simulink model "dabGAM"  (R2024b)
settings: Solver=ode23t  StartTime=0.0  StopTime=Tsim  MaxStep=dtMax  RelTol=1e-4
model workspace (MAT data in the model file):
  Cin_2 = 1e-05
  Cout_2 = 0.005
  Goff_2 = 1e-08
  L_3 = 0.001
  Lt_2 = 1e-05
  N_2 = 11
  R_1 = 0.001
  R_3 = 10
  Rds_2 = 1e-06
  Rt_2 = 0.1
  Tsim = 0.07
  Tstep = 0.035
  Vf_2 = 1e-05
  dtMax = 1e-07
  fs_2 = 50000
  order_2 = 5
libraries: nesl_utility x6, fl_lib x3, ODEsim x3
settings Model: SimulationMode=accelerator  Creator=cao2851  LastModifiedBy=cao2851
settings DataIOCC: ExternalInput=ds{1}  LoadExternalInput=on

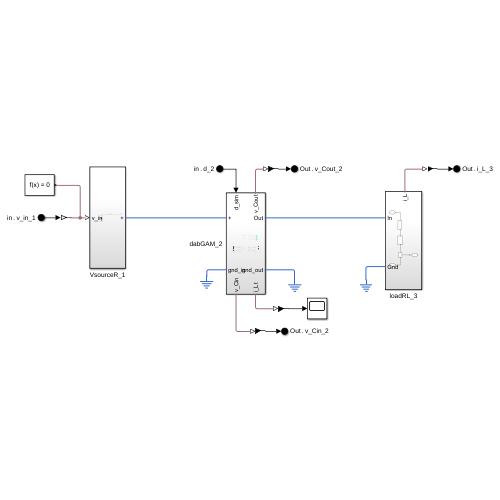
[thumbnail: Simulink's stored preview of the top-level diagram]
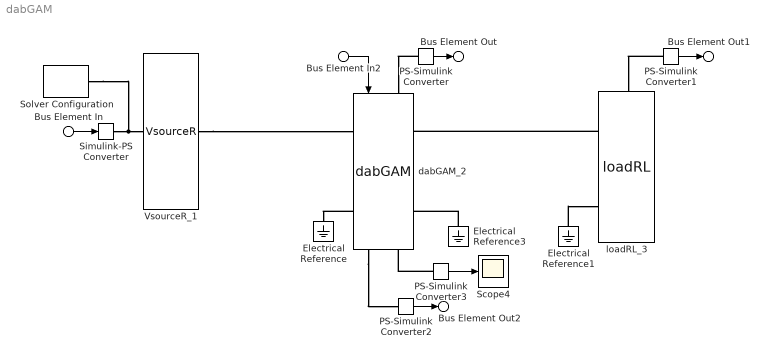
== system dabGAM ==
  Bus Element In : Inport  PortName=in  Element=v_in_1
  Bus Element In2 : Inport  PortName=in  Element=d_2
  Electrical Reference : fl_lib/Electrical/Electrical Elements/Electrical Reference
  Electrical Reference1 : fl_lib/Electrical/Electrical Elements/Electrical Reference
  Electrical Reference3 : fl_lib/Electrical/Electrical Elements/Electrical Reference
  PS-Simulink Converter{,1..3} (4 alike) : nesl_utility/PS-Simulink Converter  PhysicalDomain=network_engine_domain  SubClassName=ps_output  LeftPortType=input  RightPortType=output  PseudoPeriodic=off  Frequencies=[]  VectorFormat=inherit  Unit=inherit  AffineConversion=off
  Scope4 : Scope
  Simulink-PS Converter : nesl_utility/Simulink-PS Converter  PhysicalDomain=network_engine_domain  SubClassName=ps_input  LeftPortType=input  RightPortType=output  PseudoPeriodic=off  Frequencies=[]  NoiseDistribution=none  NoiseParameters=[]  Unit=1  AffineConversion=off  FilteringAndDerivatives=zero  SimscapeFilterOrder=1  InputFilterTimeConstant=0.001  UdotUserProvided=0
  Solver Configuration : nesl_utility/Solver Configuration  PhysicalDomain=network_engine_domain  SubClassName=solver  LeftPortType=input  RightPortType=generic  Tones=[]  Harmonics=[]  SimulateNoise=off  Profile=off  UseLocalSampling=off  EnableSwitchedLinearOptims=on  FrequencyDomain=off  UseCCode=off  RelTol=0.001  AbsTol=0.001  MinStep=1e-09  ToWorkspace=off  RevertToSquareIcSolve=off  NumHomotopyIterations=100  PhasorMode=off  PhasorModeNumHarmonics=1  ConsistencySolver=NEWTON_XTOL_AFTER_FTOL  IndexReductionMethod=DerivativeReplacement  DoDC=off  ResidualTolerance=1e-09  ConsistencyTolSource=GLOBAL  ConsistencyAbsTol=0.001  ConsistencyRelTol=0.001  ConsistencyTolFactor=1e-9  UseLocalSolver=off  LocalSolverChoice=NE_BACKWARD_EULER_ADVANCER  ResolveIndetEquations=on  FunctionEvalNumThread=1  LocalSolverSampleTime=dtMax  DoFixedCost=off  MaxNonlinIter=3  MaxModeIter=2  ComputeImpulses=off  ImpulseIterations=2  LinearAlgebra=auto  LinearAlgebraNumThread=0  EquationFormulation=NE_TIME_EF  DelaysMemoryBudget=1024  AutomaticFiltering=on  FilteringTimeConstant=0.001  PartitionStorageMethod=AS_NEEDED  PartitionMemoryBudget=1024  PartitionMethod=ROBUST  MultibodyUseLocalSolver=off  MultibodyLocalSolverChoice=ODE1  MultibodyLocalSolverSampleTime=0.001
  VsourceR_1 : ODEsim/VsourceR  SystemSampleTime=-1  VariantActivationTime=update diagram  AllowFlexibleInterface=on  Latency=0  AutoFrameSizeCalculation=off
      link override esr: R=R_1
  dabGAM_2 : ODEsim/dabGAM  SystemSampleTime=-1  VariantActivationTime=update diagram  AllowFlexibleInterface=on  Latency=0  AutoFrameSizeCalculation=off
      link override Cin: c=Cin_2
      link override Cout: C=Cout_2*10
      link override Lt: l=Lt_2  r=Rt_2
      link override S1: Rds=Rds_2  Goff=Goff_2  diode_Goff=Goff_2  diode_Ron=Rds_2  diode_Vf=Vf_2
      link override S2: Rds=Rds_2  Goff=Goff_2  diode_Goff=Goff_2  diode_Ron=Rds_2  diode_Vf=Vf_2
      link override S3: Rds=Rds_2  Goff=Goff_2  diode_Goff=Goff_2  diode_Ron=Rds_2  diode_Vf=Vf_2
      link override S4: Rds=Rds_2  Goff=Goff_2  diode_Goff=Goff_2  diode_Ron=Rds_2  diode_Vf=Vf_2
      link override S5: Rds=Rds_2  Goff=Goff_2  diode_Goff=Goff_2  diode_Ron=Rds_2  diode_Vf=Vf_2
      link override S6: Rds=Rds_2  Goff=Goff_2  diode_Goff=Goff_2  diode_Ron=Rds_2  diode_Vf=Vf_2
      link override S7: Rds=Rds_2  Goff=Goff_2  diode_Goff=Goff_2  diode_Ron=Rds_2  diode_Vf=Vf_2
      link override S8: Rds=Rds_2  Goff=Goff_2  diode_Goff=Goff_2  diode_Ron=Rds_2  diode_Vf=Vf_2
      link override Trf: n=N_2
      link override fs: Value=2*fs_2
      link override fs1: Value=2*fs_2
      settings: PortSchema="{\"entries\":[{\"content\":{\"sides\":[{\"content\":{\"connectorIds\":[\"LConn1\",\"LConn2\"]},\"type\":\"ConnectorPlacement.EquallySpacedRectSide\",\"uuid\":\"349ed430-2934-411c-8d96-d6e1ef881f7a\"},{\"content\":{\"connectorIds\":[\"RConn1\",\"RConn2\"],\"side\":\"RIGHT\"},\"type\":\"ConnectorPlacement.EquallySpacedRectSide\",\"uuid\":\"4c13ef6c-fb55-46d7-8d70-17102cf28db3\"},{\"content\":{\"connectorIds\":[\"In1\",\"LConn3\"],\"side\":\"TOP\"},\"type\":\"ConnectorPlacement.EquallySpacedRectSide\",\"uuid\":\"21058841-de4a-4ced-86ff-f9d9fda3a067\"},{\"content\":{\"connectorIds\":[\"RConn3\",\"RConn4\"],\"side\":\"BOTTOM\"},\"type\":\"ConnectorPlacement.EquallySpacedRectSide\",\"uuid\":\"f4d3d5b3-ce7a-4210-8096-b39e7c8d49a1\"}]},\"type\":\"ConnectorPlacement.EquallySpacedConnector\",\"uuid\":\"95c97b55-d26f-4f9a-9092-e1e8cc0ddd5b\"}],\"packageUris\":[\"http://schema.mathworks.com/mf0/Connector/R2020b\"],\"version\":\"1.0\"}"
  loadRL_3 : ODEsim/loadRL  SystemSampleTime=-1  VariantActivationTime=update diagram  AllowFlexibleInterface=on  Latency=0  AutoFrameSizeCalculation=off
      link override Lload: l=L_3
      link override Rload: R=R_3
      settings: PortSchema="{\"entries\":[{\"content\":{\"sides\":[{\"content\":{\"connectorIds\":[\"LConn1\",\"LConn2\"]},\"type\":\"ConnectorPlacement.EquallySpacedRectSide\",\"uuid\":\"06c3c841-7f27-414f-b368-a176494b6f9d\"},{\"content\":{\"side\":\"RIGHT\"},\"type\":\"ConnectorPlacement.EquallySpacedRectSide\",\"uuid\":\"1b123208-a0a4-432d-8d9c-871fed45b507\"},{\"content\":{\"connectorIds\":[\"LConn3\"],\"side\":\"TOP\"},\"type\":\"ConnectorPlacement.EquallySpacedRectSide\",\"uuid\":\"cfe0dd68-fe1a-447a-9562-3abbfb037eea\"}]},\"type\":\"ConnectorPlacement.EquallySpacedConnector\",\"uuid\":\"2a5dcc2a-148a-4bfc-a97a-46b06b110d1b\"}],\"packageUris\":[\"http://schema.mathworks.com/mf0/Connector/R2020b\"],\"version\":\"1.0\"}"
  Bus Element Out : Outport  PortName=Out  Element=v_Cout_2
  Bus Element Out2 : Outport  PortName=Out  Element=v_Cin_2
  Bus Element Out1 : Outport  PortName=Out  Element=i_L_3
  wires:
  Bus Element In/1 -> Simulink-PS Converter/1
  Bus Element In2/1 -> dabGAM_2/1
  PS-Simulink Converter1/1 -> Bus Element Out1/1
  PS-Simulink Converter/1 -> Bus Element Out/1
  PS-Simulink Converter2/1 -> Bus Element Out2/1
  PS-Simulink Converter3/1 -> Scope4/1
  connections:
  dabGAM_2/LConn2 -- Electrical Reference/LConn1
  PS-Simulink Converter/LConn1 -- dabGAM_2/LConn3
  dabGAM_2/RConn3 -- PS-Simulink Converter2/LConn1
  VsourceR_1/RConn1 -- dabGAM_2/LConn1
  Electrical Reference3/LConn1 -- dabGAM_2/RConn2
  Simulink-PS Converter/RConn1 -- Solver Configuration/RConn1 -- VsourceR_1/LConn1
  loadRL_3/LConn1 -- dabGAM_2/RConn1
  Electrical Reference1/LConn1 -- loadRL_3/LConn2
  PS-Simulink Converter1/LConn1 -- loadRL_3/LConn3
  PS-Simulink Converter3/LConn1 -- dabGAM_2/RConn4
